simulink model "crossARINC_out"  (R2021b)
settings: Solver=FixedStepDiscrete  StartTime=0.0  StopTime=inf  RelTol=1e-3
undefined symbols (not defined in the file): IO682
libraries: speedgoatlib_IO682 x9
settings Model: Creator=ACH  LastModifiedBy=angel
settings SolverCC: ConcurrentTasks=on  PositivePriorityOrder=on
settings OptimizationCC: BlockReduction=off  OptimizeBlockIOStorage=off
settings DebuggingCC: TasksWithSamePriorityMsg=none
settings HardwareCC: ProdBitPerLong=64  ProdLongLongMode=on  ProdHWDeviceType=Intel->x86-64 (Linux 64)
settings RTWCC: Description=Simulink Real-Time  SystemTargetFile=slrealtime.tlc  TemplateMakefile=slrealtime_default_tmf  Toolchain=Simulink Real-Time Toolchain  BuildConfiguration=Faster Runs  CodeExecutionProfiling=on  TargetLang=C++
settings SimulinkRealTimeTargetCC: UseGCCFastMath=on

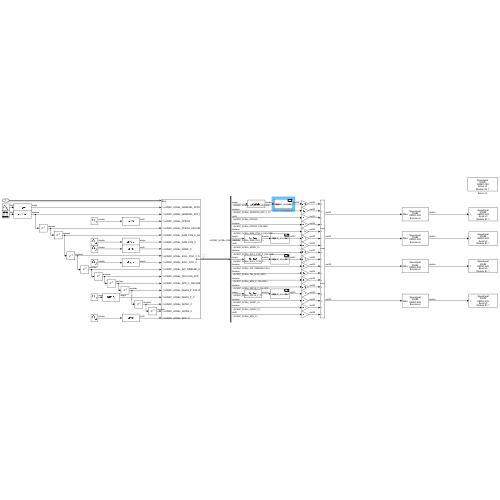
[thumbnail: Simulink's stored preview of the top-level diagram]
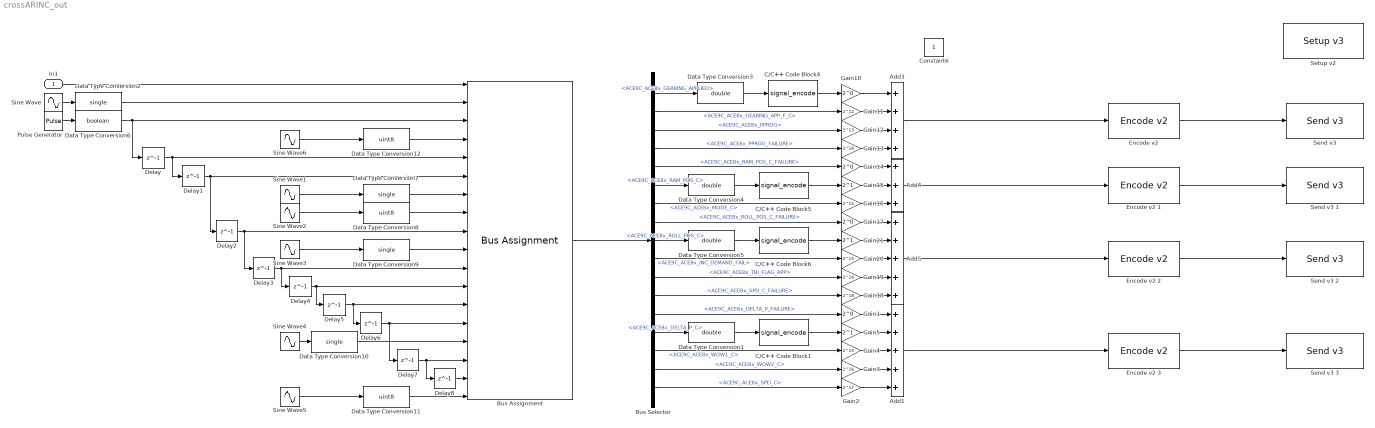
== system crossARINC_out ==
  In1 : Inport  OutDataTypeStr=Bus: ACE9C_ACE8x_9C
  Add1 : Sum  Inputs=+++++
  Add3 : Sum  Inputs=++++
  Add4 : Sum  Inputs=+++
  Add5 : Sum  Inputs=+++++
  Bus Assignment : BusAssignment  AssignedSignals=ACE9C_ACE8x_GEARING_APPLIED,ACE9C_ACE8x_GEARING_APP_F_C,ACE9C_ACE8x_PPROG,ACE9C_ACE8x_PPROG_FAILURE,ACE9C_ACE8x_RAM_POS_C_FAILURE,ACE9C_ACE8x_RAM_POS_C,ACE9C_ACE8x_MODE_C,ACE9C_ACE8x_ROLL_POS_C_FAILURE,ACE9C_ACE8x_ROLL_POS_C,ACE9C_ACE8x_INC_DEMAND_FAIL,ACE9C_ACE8x_TBI_FLAG_APP,ACE9C_ACE8x_SPD_C_FAILURE,ACE9C_ACE8x_DELTA_P_FAILURE,ACE9C_ACE8x_DELTA_P_C,ACE9C_ACE8x_WOW1_C,ACE9C_ACE8x_WOW2_C,ACE9C_ACE8x_SPD_C
  Bus Selector : BusSelector  OutputSignals=ACE9C_ACE8x_GEARING_APPLIED,ACE9C_ACE8x_GEARING_APP_F_C,ACE9C_ACE8x_PPROG,ACE9C_ACE8x_PPROG_FAILURE,ACE9C_ACE8x_RAM_POS_C_FAILURE,ACE9C_ACE8x_RAM_POS_C,ACE9C_ACE8x_MODE_C,ACE9C_ACE8x_ROLL_POS_C_FAILURE,ACE9C_ACE8x_ROLL_POS_C,ACE9C_ACE8x_INC_DEMAND_FAIL,ACE9C_ACE8x_TBI_FLAG_APP,ACE9C_ACE8x_SPD_C_FAILURE,ACE9C_ACE8x_DELTA_P_FAILURE,ACE9C_ACE8x_DELTA_P_C,ACE9C_ACE8x_WOW1_C,ACE9C_ACE8x_WOW2_C,ACE9C_ACE8x_SPD_C
  C/C++ Code Block1 : S-Function  FunctionName=signal_encode  Parameters=2.808E-2,0,boolean(1),boolean(0),uint32(14)  SFunctionModules=signal_encode_wrapper  SFunctionDeploymentMode=off  EnableBusSupport=off  mask(S-Function Builder){}
      mask help: Simulink:masks:SFunctionBuilder_MD
      mask init:
      | val = [[.9  0.75 0.75 1 1 .9 .9 1]',[1 1 0.75 0.75 .9 .9 1 .9]'];try , sys = get_param(gcb,'SfunBuilderFcnName');if isempty(sys), sys = get_param(gcb,'FunctionName'); end,catch, sys = get_param(gcb,'FunctionName'); end
      settings: CopyFcn=set_param(gcbh,'LinkStatus','none')  OpenFcn=sfunctionwizard(gcbh)
      mask Display:
      | plot(val(:,1),val(:,2))
      | disp(sys)
      | port_label('input',1,'data')
      | port_label('output',1,'out')
  C/C++ Code Block4 : S-Function  FunctionName=signal_encode  Parameters=6.10501E-5,0.2,boolean(0),boolean(0),uint32(12)  SFunctionModules=signal_encode_wrapper  SFunctionDeploymentMode=off  EnableBusSupport=off  mask(S-Function Builder){}
      mask help: Simulink:masks:SFunctionBuilder_MD
      mask init: same as crossARINC_out/C/C++ Code Block1
      settings: CopyFcn=set_param(gcbh,'LinkStatus','none')  OpenFcn=sfunctionwizard(gcbh)
      mask Display: plot(val(:,1),val(:,2)),disp(sys),port_label('input',1,'data'),port_label('output',1,'out')
  C/C++ Code Block5 : S-Function  FunctionName=signal_encode  Parameters=3.2963E-3,0,boolean(1),boolean(0),uint32(14)  SFunctionModules=signal_encode_wrapper  SFunctionDeploymentMode=off  EnableBusSupport=off  mask(S-Function Builder){}
      mask help: Simulink:masks:SFunctionBuilder_MD
      mask init: same as crossARINC_out/C/C++ Code Block1
      settings: CopyFcn=set_param(gcbh,'LinkStatus','none')  OpenFcn=sfunctionwizard(gcbh)
      mask Display: plot(val(:,1),val(:,2)),disp(sys),port_label('input',1,'data'),port_label('output',1,'out')
  C/C++ Code Block6 : S-Function  FunctionName=signal_encode  Parameters=9.76682E-3,0,boolean(1),boolean(0),uint32(14)  SFunctionModules=signal_encode_wrapper  SFunctionDeploymentMode=off  EnableBusSupport=off  mask(S-Function Builder){}
      mask help: Simulink:masks:SFunctionBuilder_MD
      mask init: same as crossARINC_out/C/C++ Code Block1
      settings: CopyFcn=set_param(gcbh,'LinkStatus','none')  OpenFcn=sfunctionwizard(gcbh)
      mask Display:
      | plot(val(:,1),val(:,2))
      | disp(sys)
      | port_label('input',1,'data')
      | port_label('output',1,'out')
  Data Type Conversion{1,3..5} (4 alike) : DataTypeConversion  OutDataTypeStr=double
  Data Type Conversion{2,7,9..10} (4 alike) : DataTypeConversion  OutDataTypeStr=single
  Data Type Conversion11 : DataTypeConversion  OutDataTypeStr=uint8
  Data Type Conversion12 : DataTypeConversion  OutDataTypeStr=uint8
  Data Type Conversion6 : DataTypeConversion  OutDataTypeStr=boolean
  Data Type Conversion8 : DataTypeConversion  OutDataTypeStr=uint8
  Delay{,1..8} (9 alike) : Delay  DelayLength=1
  "Encode v2 " : speedgoatlib_IO682/Encode v2   parMode=Custom Data Type  parLabel=[55]  parDataType=[0]  parResolution=[1]  parBits=[19]  parSdi=[0]  parSsm=[-1]  parCustomDataType=Raw  parDataLSB=11  parDataMSB=31  parBitPosition=[9, 31]  parScaleBNR=1  parExponent=8  parMantissa=14  parEnSSM=off
      settings: SourceProductName=Simulink Real-Time: Speedgoat I/O Blockset
  Encode v2 1 : speedgoatlib_IO682/Encode v2   parMode=Custom Data Type  parLabel=[112]  parDataType=[0]  parResolution=[1]  parBits=[19]  parSdi=[0]  parSsm=[-1]  parCustomDataType=Raw  parDataLSB=11  parDataMSB=31  parBitPosition=[9, 31]  parScaleBNR=1  parExponent=8  parMantissa=14  parEnSSM=off
      settings: SourceProductName=Simulink Real-Time: Speedgoat I/O Blockset
  Encode v2 2 : speedgoatlib_IO682/Encode v2   parMode=Custom Data Type  parLabel=[163]  parDataType=[0]  parResolution=[1]  parBits=[19]  parSdi=[0]  parSsm=[-1]  parCustomDataType=Raw  parDataLSB=11  parDataMSB=31  parBitPosition=[9, 31]  parScaleBNR=1  parExponent=8  parMantissa=14  parEnSSM=off
      settings: SourceProductName=Simulink Real-Time: Speedgoat I/O Blockset
  Encode v2 3 : speedgoatlib_IO682/Encode v2   parMode=Custom Data Type  parLabel=[231]  parDataType=[0]  parResolution=[1]  parBits=[19]  parSdi=[0]  parSsm=[-1]  parCustomDataType=Raw  parDataLSB=11  parDataMSB=31  parBitPosition=[9, 31]  parScaleBNR=1  parExponent=8  parMantissa=14  parEnSSM=off
      settings: SourceProductName=Simulink Real-Time: Speedgoat I/O Blockset
  Gain{1,10,14,17} (4 alike) : Gain  Gain=2^0  OutDataTypeStr=uint32
  Gain11 : Gain  Gain=2^12  OutDataTypeStr=uint32
  Gain12 : Gain  Gain=2^13  OutDataTypeStr=uint32
  Gain13 : Gain  Gain=2^18  OutDataTypeStr=uint32
  Gain15 : Gain  Gain=2^1  OutDataTypeStr=uint32
  Gain16 : Gain  Gain=2^15  OutDataTypeStr=uint32
  Gain18 : Gain  Gain=2^18  OutDataTypeStr=uint32
  Gain19 : Gain  Gain=2^16  OutDataTypeStr=uint32
  Gain2 : Gain  Gain=2^17  OutDataTypeStr=uint32
  Gain20 : Gain  Gain=2^15  OutDataTypeStr=uint32
  Gain21 : Gain  Gain=2^1  OutDataTypeStr=uint32
  Gain3 : Gain  Gain=2^16  OutDataTypeStr=uint32
  Gain4 : Gain  Gain=2^15  OutDataTypeStr=uint32
  Gain5 : Gain  Gain=2^1  OutDataTypeStr=uint32
  Pulse Generator : DiscretePulseGenerator  Period=125  PulseWidth=25  SampleTime=0.008
  Send v3 {,1..3} (4 alike) : speedgoatlib_IO682/Send v3   parModuleId=1  parChannel=1  parSampleTime=0.008
      settings: SourceProductName=Simulink Real-Time: Speedgoat I/O Blockset
  "Setup v2 " : speedgoatlib_IO682/Setup v3   parModuleId=1  parBoardVariant=IO682-16-16  parPciSlot=-1  parTimerCount=4000*8  parChannelMode=Manual  parInBitRate1=100000  parInBufferMode1=Individual  parInEnable1=on  parInParity1=off  parInInternalWrap1=off  parInBitRate2=100000  parInBufferMode2=Individual  parInEnable2=on  parInParity2=on  parInInternalWrap2=off  parInBitRate3=100000  parInBufferMode3=Individual  parInEnable3=on  parInParity3=on  parInInternalWrap3=off  parInBitRate4=100000  parInBufferMode4=Individual  parInEnable4=on  parInParity4=on  parInInternalWrap4=off  parInBitRate5=100000  parInBufferMode5=Individual  parInEnable5=on  parInParity5=on  parInInternalWrap5=off  parInBitRate6=100000  parInBufferMode6=Individual  parInEnable6=on  parInParity6=on  parInInternalWrap6=off  parInBitRate7=100000  parInBufferMode7=Individual  parInEnable7=on  parInParity7=on  parInInternalWrap7=off  parInBitRate8=100000  parInBufferMode8=Individual  parInEnable8=on  parInParity8=on  parInInternalWrap8=off  parInBitRate9=100000  parInBufferMode9=Individual  parInEnable9=on  parInParity9=on  parInInternalWrap9=off  parInBitRate10=100000  parInBufferMode10=Individual  parInEnable10=on  parInParity10=on  parInInternalWrap10=off  parInBitRate11=100000  parInBufferMode11=Individual  parInEnable11=on  parInParity11=on  parInInternalWrap11=off  parInBitRate12=100000  parInBufferMode12=Individual  parInEnable12=on  parInParity12=on  parInInternalWrap12=off  parInBitRate13=100000  parInBufferMode13=Individual  parInEnable13=on  parInParity13=on  parInInternalWrap13=off  parInBitRate14=100000  parInBufferMode14=Individual  parInEnable14=on  parInParity14=on  parInInternalWrap14=off  parInBitRate15=100000  parInBufferMode15=Individual  parInEnable15=on  parInParity15=on  parInInternalWrap15=off  parInBitRate16=100000  parInBufferMode16=Individual  parInEnable16=on  parInParity16=on  parInInternalWrap16=off  parOutBitRate1=100000  parOutParity1=Odd  parOutProtocolError1=None  parOutEnable1=on  parOutBitRate2=100000  parOutParity2=Odd  parOutProtocolError2=None  parOutEnable2=on  parOutBitRate3=100000  parOutParity3=Odd  parOutProtocolError3=None  parOutEnable3=on  parOutBitRate4=100000  parOutParity4=Odd  parOutProtocolError4=None  parOutEnable4=on  parOutBitRate5=100000  parOutParity5=Odd  parOutProtocolError5=None  parOutEnable5=on  parOutBitRate6=100000  parOutParity6=Odd  parOutProtocolError6=None  parOutEnable6=on  parOutBitRate7=100000  parOutParity7=Odd  parOutProtocolError7=None  parOutEnable7=on  parOutBitRate8=100000  parOutParity8=Odd  parOutProtocolError8=None  parOutEnable8=on  parOutBitRate9=100000  parOutParity9=Odd  parOutProtocolError9=None  parOutEnable9=on  parOutBitRate10=100000  parOutParity10=Odd  parOutProtocolError10=None  parOutEnable10=on  parOutBitRate11=100000  parOutParity11=Odd  parOutProtocolError11=None  parOutEnable11=on  parOutBitRate12=100000  parOutParity12=Odd  parOutProtocolError12=None  parOutEnable12=on  parOutBitRate13=100000  parOutParity13=Odd  parOutProtocolError13=None  parOutEnable13=on  parOutBitRate14=100000  parOutParity14=Odd  parOutProtocolError14=None  parOutEnable14=on  parOutBitRate15=100000  parOutParity15=Odd  parOutProtocolError15=None  parOutEnable15=on  parOutBitRate16=100000  parOutParity16=Odd  parOutProtocolError16=None  parOutEnable16=on  parChConfigFile=''  parScheduleMode=Manual  parScheduledMsgConfigFile=''  parHwDeviceId=hex2dec('0830')  parTimeSource=Internal timer  parChInConfig=[158 8 7 8 1;158 8 7 7 1;158 8 7 7 1;158 8 7 7 1;158 8 7 7 1;158 8 7 7 1;158 8 7 7 1;158 8 7 7 1;158 8 7 7 1;158 8 7 7 1;158 8 7 7 1;158 8 7 7 1;158 8 7 7 1;158 8 7 7 1;158 8 7 7 1;158 8 7 7 1]  parChOutConfig=[158 0 4 7;158 0 4 7;158 0 4 7;158 0 4 7;158 0 4 7;158 0 4 7;158 0 4 7;158 0 4 7;158 0 4 7;158 0 4 7;158 0 4 7;158 0 4 7;158 0 4 7;158 0 4 7;158 0 4 7;158 0 4 7]  parScheduledMessages=0
      settings: SourceProductName=Speedgoat I/O Blockset
  Sine Wave : Sin  Amplitude=(0.45-0.2)/2*0.99  Bias=0.2+(0.45-0.2)/2  Frequency=2*pi  SampleTime=0.008
  Sine Wave1 : Sin  Amplitude=27*0.99  Frequency=2*pi  SampleTime=0.008
  Sine Wave2 : Sin  Amplitude=3.5  Bias=4  Frequency=2*pi  SampleTime=0.008
  Sine Wave3 : Sin  Amplitude=80*0.99  Frequency=2*pi  SampleTime=0.008
  Sine Wave4 : Sin  Amplitude=230*0.99  Frequency=2*pi  SampleTime=0.008
  Sine Wave5 : Sin  Amplitude=1.5  Bias=2  Frequency=2*pi  SampleTime=0.008
  Sine Wave6 : Sin  Amplitude=7.5  Bias=8  Frequency=2*pi  SampleTime=0.008
  Constant6 : Constant  IOType=siggen
  wires:
  Add3/1 -> "Encode v2 "/1
  "Encode v2 "/1 -> "Send v3 "/1
  Encode v2 1/1 -> Send v3 1/1
  Add4/1 -> Encode v2 1/1
  Encode v2 2/1 -> Send v3 2/1
  Encode v2 3/1 -> Send v3 3/1
  Bus Assignment/1 -> Bus Selector/1
  In1/1 -> Bus Assignment/1
  Pulse Generator/1 -> Data Type Conversion6/1
  Delay/1 -> Delay1/1, Bus Assignment/5
  Delay2/1 -> Delay3/1, Bus Assignment/9
  Delay3/1 -> Delay4/1, Bus Assignment/11
  Delay4/1 -> Delay5/1, Bus Assignment/12
  Delay5/1 -> Delay6/1, Bus Assignment/13
  Delay6/1 -> Delay7/1, Bus Assignment/14
  Data Type Conversion10/1 -> Bus Assignment/15
  Data Type Conversion8/1 -> Bus Assignment/8
  Delay1/1 -> Delay2/1, Bus Assignment/6
  Data Type Conversion7/1 -> Bus Assignment/7
  Bus Selector/1 -> Data Type Conversion3/1  "<ACE9C_ACE8x_GEARING_APPLIED>"
  Data Type Conversion3/1 -> C/C++ Code Block4/1
  C/C++ Code Block4/1 -> Gain10/1
  Gain10/1 -> Add3/1
  Gain11/1 -> Add3/2
  Bus Selector/2 -> Gain11/1  "<ACE9C_ACE8x_GEARING_APP_F_C>"
  Bus Selector/3 -> Gain12/1  "<ACE9C_ACE8x_PPROG>"
  Gain12/1 -> Add3/3
  Gain13/1 -> Add3/4
  Bus Selector/4 -> Gain13/1  "<ACE9C_ACE8x_PPROG_FAILURE>"
  Bus Selector/5 -> Gain14/1  "<ACE9C_ACE8x_RAM_POS_C_FAILURE>"
  Gain14/1 -> Add4/1
  Data Type Conversion4/1 -> C/C++ Code Block5/1
  Bus Selector/6 -> Data Type Conversion4/1  "<ACE9C_ACE8x_RAM_POS_C>"
  C/C++ Code Block5/1 -> Gain15/1
  Gain15/1 -> Add4/2
  Bus Selector/7 -> Gain16/1  "<ACE9C_ACE8x_MODE_C>"
  Gain16/1 -> Add4/3
  Bus Selector/8 -> Gain17/1  "<ACE9C_ACE8x_ROLL_POS_C_FAILURE>"
  Bus Selector/9 -> Data Type Conversion5/1  "<ACE9C_ACE8x_ROLL_POS_C>"
  Bus Selector/10 -> Gain20/1  "<ACE9C_ACE8x_INC_DEMAND_FAIL>"
  Bus Selector/11 -> Gain19/1  "<ACE9C_ACE8x_TBI_FLAG_APP>"
  Bus Selector/12 -> Gain18/1  "<ACE9C_ACE8x_SPD_C_FAILURE>"
  Gain17/1 -> Add5/1
  Gain18/1 -> Add5/5
  Gain19/1 -> Add5/4
  Gain20/1 -> Add5/3
  Gain21/1 -> Add5/2
  C/C++ Code Block6/1 -> Gain21/1
  Data Type Conversion5/1 -> C/C++ Code Block6/1
  Add5/1 -> Encode v2 2/1
  Add1/1 -> Encode v2 3/1
  Data Type Conversion1/1 -> C/C++ Code Block1/1
  C/C++ Code Block1/1 -> Gain5/1
  Gain5/1 -> Add1/2
  Gain4/1 -> Add1/3
  Gain3/1 -> Add1/4
  Gain2/1 -> Add1/5
  Gain1/1 -> Add1/1
  Bus Selector/17 -> Gain2/1  "<ACE9C_ACE8x_SPD_C>"
  Bus Selector/16 -> Gain3/1  "<ACE9C_ACE8x_WOW2_C>"
  Bus Selector/15 -> Gain4/1  "<ACE9C_ACE8x_WOW1_C>"
  Bus Selector/14 -> Data Type Conversion1/1  "<ACE9C_ACE8x_DELTA_P_C>"
  Bus Selector/13 -> Gain1/1  "<ACE9C_ACE8x_DELTA_P_FAILURE>"
  Data Type Conversion2/1 -> Bus Assignment/2
  Sine Wave/1 -> Data Type Conversion2/1
  Data Type Conversion6/1 -> Bus Assignment/3, Delay/1
  Delay7/1 -> Delay8/1, Bus Assignment/16
  Delay8/1 -> Bus Assignment/17
  Sine Wave1/1 -> Data Type Conversion7/1
  Sine Wave2/1 -> Data Type Conversion8/1
  Sine Wave3/1 -> Data Type Conversion9/1
  Data Type Conversion9/1 -> Bus Assignment/10
  Sine Wave4/1 -> Data Type Conversion10/1
  Data Type Conversion11/1 -> Bus Assignment/18
  Sine Wave5/1 -> Data Type Conversion11/1
  Sine Wave6/1 -> Data Type Conversion12/1
  Data Type Conversion12/1 -> Bus Assignment/4
